simulink model "s1"  (R2016b)
settings: Solver=VariableStepAuto  StartTime=0.0  StopTime=10.0  RelTol=1e-3
settings Model: Creator=fabia  LastModifiedBy=fabia

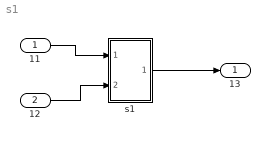
== system s1 ==
  11 : Inport
  12 : Inport  Port=2
  "s1 " : Subsystem
  13 : Outport
  wires:
  11/1 -> "s1 "/1(In1)
  12/1 -> "s1 "/2(In2)
  "s1 "/1(Out1) -> 13/1

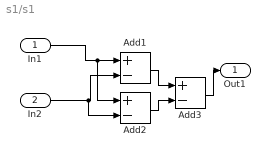
== system s1/s1  ==
  In1 : Inport
  In2 : Inport  Port=2
  Add1 : Sum  Inputs=+-
  Add2 : Sum  Inputs=+-
  Add3 : Sum  Inputs=+-
  Out1 : Outport
  wires:
  In1/1 -> Add2/1, Add1/1
  In2/1 -> Add2/2, Add1/2
  Add3/1 -> Out1/1
  Add1/1 -> Add3/1
  Add2/1 -> Add3/2
